simulink model "DacTinhCo"  (R2019a)
settings: Solver=VariableStepAuto  StartTime=0.0  StopTime=2.0  RelTol=1e-3
values from neighbouring files (symbols this model uses):
  Raf = 1    [thamSoDongCo.m]
  RafEnable = 0    [DacTinhCoThayDoiVa.m]    (also in DacTinhThayDoiKPhi.m; DacTinhThayDoiRaf.m = 1; thamSoDongCo.m)
  TL = 100    [DacTinhHamDongNang.m]    (also in DacTinhHamNguoc.m = 75)
  Va = 240    [thamSoDongCo.m]
  Vf = 150    [thamSoDongCo.m]
libraries: powerlib x6
settings Model: Creator=Admin  LastModifiedBy=Phong

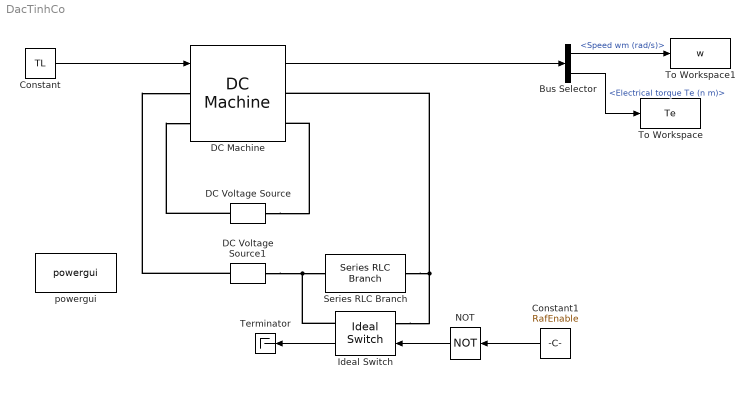
== system DacTinhCo ==
  Bus Selector : BusSelector  OutputSignals=Speed wm (rad/s),Electrical torque Te (n m)
  Constant : Constant  Value=TL
  Constant1 : Constant  Value=RafEnable
  DC Machine : powerlib/Machines/DC Machine  PresetModel=No  MechanicalLoad=Torque TL  FieldType=Wound  ShowDetailedParameters=on  MeasurementBus=off  RLa=[0.78 0.016]  RLf=[150 112.5]  Laf=1.234  MachineConstant=Torque constant (N.m/A)  Ke=1.8  Kt=1.8  J=0.25  Bm=0.01  Tf=0  w0=0  Ifinit=0  TsPowergui=0  TsBlock=-1
      settings: SourceProductName=Simscape Electrical
  DC Voltage Source : powerlib/Electrical Sources/DC Voltage Source  Amplitude=Vf  Measurements=None
      settings: SourceProductName=Simscape Electrical
  DC Voltage Source1 : powerlib/Electrical Sources/DC Voltage Source  Amplitude=Va  Measurements=None
      settings: SourceProductName=Simscape Electrical
  Ideal Switch : powerlib/Power Electronics/Ideal Switch  Ron=0  Lon=0  IC=0  Rs=0  Cs=0  Measurements=on
      settings: SourceProductName=Simscape Electrical
  NOT : Logic  Operator=NOT  IconShape=distinctive  AllPortsSameDT=off  OutDataTypeStr=boolean
  Series RLC Branch : powerlib/Elements/Series RLC Branch  LConnTagsString=__new0  RConnTagsString=__new0  BranchType=R  Resistance=Raf  Inductance=1e-3  SetiL0=off  InitialCurrent=0  Capacitance=1e-6  Setx0=off  InitialVoltage=0  Measurements=None
      settings: SourceProductName=Simscape Electrical
  Terminator : Terminator
  To Workspace : ToWorkspace  VariableName=Te  SampleTime=-1
  To Workspace1 : ToWorkspace  VariableName=w  SampleTime=-1
  powergui : powerlib/powergui  Priority=1  SimulationMode=Continuous  SampleTime=50e-6  frequency=60  Iterations=50  frequencyindice=0  Pbase=100e6  ErrMax=1e-4  UnitsV=kV  UnitsW=MW  buscounter=0  FunctionMessages=off  echomessages=off  EnableUseOfTLC=off  CurrentSourceSwitches=off  DisableSnubberDevices=off  DisableRonSwitches=off  DisableVfSwitches=off  DisplayEquations=off  AutomaticDiscreteSolvers=off  SolverType=Tustin/Backward Euler (TBE)  Interpol=off  ExternalGateDelay=off  methode=off  Ts=100  x0status=blocks  SPID=on  SwTol=0  HookPort=off  NonlinearTolerance=0  nMaxIteration=15  ContinueOnMaxIteration=off  RestoreLinks=warning  ResistiveCurrentMeasurement=off  Frange=[0:2:500]  Ylog=off  Xlog=on  ShowGrid=off  save=off  variable=ZData  structure=0  ZoomFFT=off  StartTime=0.0  cycles=1  DisplayStyle=1  fundamental=60  FreqAxis=off  MaxFrequency=1000  frequencyindicesteady=1  RmsSteady=1  display=off
      settings: SourceProductName=Simscape Electrical
  wires:
  Constant/1 -> DC Machine/1
  DC Machine/1 -> Bus Selector/1
  Bus Selector/1 -> To Workspace1/1  "<Speed wm (rad/s)>"
  Bus Selector/2 -> To Workspace/1  "<Electrical torque Te (n m)>"
  NOT/1 -> Ideal Switch/1
  Constant1/1 -> NOT/1
  Ideal Switch/1 -> Terminator/1
  connections:
  DC Voltage Source/LConn1 -- DC Machine/RConn2
  DC Voltage Source1/RConn1 -- DC Machine/LConn1
  DC Voltage Source/RConn1 -- DC Machine/LConn2
  DC Voltage Source1/LConn1 -- Ideal Switch/RConn1 -- Series RLC Branch/LConn1
  Series RLC Branch/RConn1 -- Ideal Switch/LConn1 -- DC Machine/RConn1
